simulink model "pmsm_FOC"  (R2018a)
settings: Solver=ode3  StartTime=0.0  StopTime=20  FixedStep=Ts  RelTol=1e-3  EnableMultiTasking=on
InitFcn:
  | % PMSM电机模型参数
  | P=8;
  | Ld=4.63e-4;
  | Lq=4.63e-4;
  | Flux_m=7.07e-3;
  | R=0.608;
  | J = 1.87e-3;
  | Beta=0;% 阻尼系数   (N s/m)
  | 
  | % 离散时间间隔
  | Ts = 1e-4;
  | 
  | % 观测器参数
  | w = 1000;
  | b = 500;
  | T = 0.01;
  | 
  | % TD微分跟踪器参数
  | tr=2000;
  | th = Ts*3;
  | 
  | % DOB转动惯量在线辨识参数
  | Jn = J
  | lamuda = 200
  | Te = 0.2
libraries: simulink x2, fuzblock x1
settings Model: Creator=www  LastModifiedBy=SPRain
settings SolverCC: AutoInsertRateTranBlk=on
settings DataIOCC: LimitDataPoints=on  SaveFormat=Array
settings OptimizationCC: ExpressionDepthLimit=2147483647  LifeSpan=inf
settings DebuggingCC: UnderspecifiedInitializationDetection=Classic  MergeDetectMultiDrivingBlocksExec=none  SolverPrmCheckMsg=warning  FcnCallInpInsideContextMsg=warning  StateNameClashWarn=warning  SFUnexpectedBacktrackingDiag=warning  SFNoUnconditionalDefaultTransitionDiag=warning  SFExecutionAtInitializationDiag=none
settings HardwareCC: ProdBitPerPointer=32  ProdBitPerSizeT=32  ProdBitPerPtrDiffT=32  ProdLargestAtomicFloat=None  ProdIntDivRoundTo=Undefined  ProdEndianess=Unspecified  ProdWordSize=32  ProdHWDeviceType=32-bit Generic
settings ModelReferenceCC: PropagateSignalLabelsOutOfModel=off
settings CodeAppCC: StateflowObjectComments=on
settings GRTTargetCC: TargetLangStandard=C89/C90 (ANSI)  GeneratePreprocessorConditionals=Disable all  CombineOutputUpdateFcns=off  GRTInterface=on
settings ConfigComp: CovMetricSettings=dw  CovHtmlReporting=on  CovSaveCumulativeToWorkspaceVar=on  CovSaveSingleToWorkspaceVar=on  CovExternalEMLEnable=off  CovSFcnEnable=off

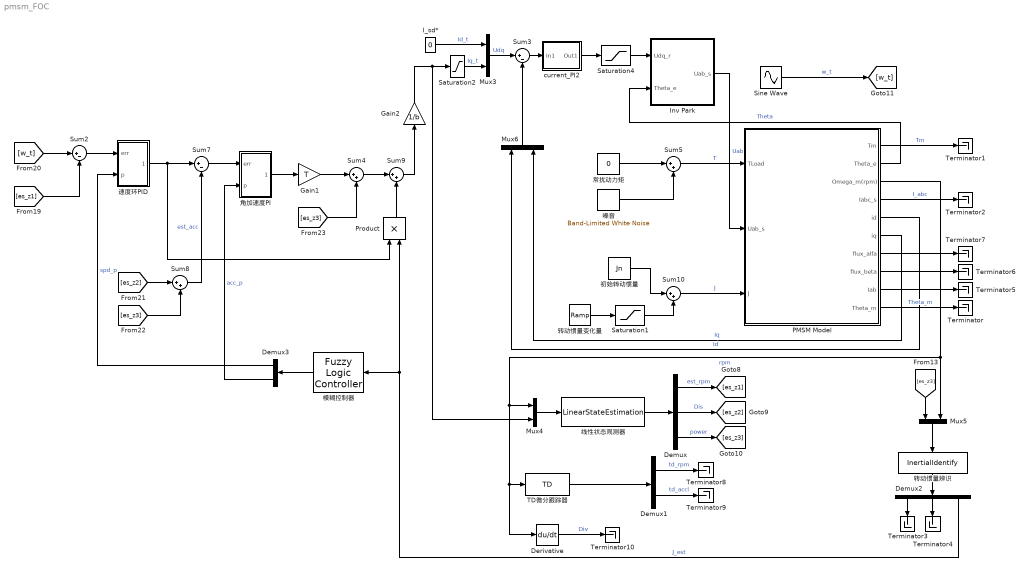
== system pmsm_FOC ==
  Demux : Demux  Outputs=3
  Demux1 : Demux  Outputs=2
  Demux2 : Demux  Outputs=3
  Demux3 : Demux  Outputs=2
  Derivative : Derivative
  Gain1 : Gain  Gain=T
  Gain2 : Gain  Gain=1/b
  I_sd* : Constant  Value=0
  Inv Park : Subsystem
  Mux{3..6} (4 alike) : Mux  Inputs=2
  PMSM Model : Subsystem
  Product : Product
  Saturation1 : Saturate  UpperLimit=0.02  LowerLimit=0
  Saturation2 : Saturate  UpperLimit=100  LowerLimit=-100
  Saturation4 : Saturate  UpperLimit=100  LowerLimit=-100
  Sine Wave : Sin  Amplitude=50  Frequency=5*pi  SampleTime=0
  Sum10 : Sum  Inputs=|++  SaturateOnIntegerOverflow=on  InputSameDT=on  OutDataTypeStr=Inherit: Same as first input
  Sum2 : Sum  Inputs=|+-
  Sum3 : Sum  Inputs=|+-
  Sum4 : Sum  Inputs=|++
  Sum5 : Sum  Inputs=|++  SaturateOnIntegerOverflow=on  InputSameDT=on  OutDataTypeStr=Inherit: Same as first input
  Sum7 : Sum  Inputs=|+-
  Sum8 : Sum  Inputs=|++  SaturateOnIntegerOverflow=on  InputSameDT=on  OutDataTypeStr=Inherit: Same as first input
  Sum9 : Sum  Inputs=|++
  TD微分跟踪器 : S-Function  FunctionName=TD  Parameters=tr,th,Ts  SFunctionDeploymentMode=off  EnableBusSupport=off
  Terminator{,1..10} (11 alike) : Terminator
  current_PI2 : Subsystem
  初始转动惯量 : Constant  Value=Jn
  噪音 : simulink/Sources/Band-Limited White Noise  Cov=[0.00001]  Ts=0.1  seed=[23341]
  常扰动力矩 : Constant  Value=0
  模糊控制器 : fuzblock/Fuzzy Logic  Controller  FIS='J_Fuzzy.fis'  OutputSampleNumber=101  DataType=double  FuzzifiedInputs=off  RuleFiringStrengths=off  RuleOutputs=off  AggregatedOutputs=off  SimulateUsing=Interpreted execution  OutOfRangeInputValueMessage=warning  NoRuleFiredMessage=warning  EmptyOutputFuzzySetMessage=warning
  线性状态观测器 : S-Function  FunctionName=LinearStateEstimation  Parameters=w,b,Ts,T  SFunctionDeploymentMode=off  EnableBusSupport=off
  角加速度PI : Subsystem
  转动惯量变化量 : simulink/Sources/Ramp  slope=0.002  start=5  InitialOutput=0
  转动惯量辨识 : S-Function  FunctionName=InertialIdentify  Parameters=lamuda,Ts,Te,Jn  SFunctionDeploymentMode=off  EnableBusSupport=off
  速度环PID : Subsystem
  wires:
  Saturation4/1 -> Inv Park/1(Udq_r)
  Inv Park/1(Uab_s) -> PMSM Model/2(Uab_s)  "Uab"
  I_sd*/1 -> Mux3/1  "Id_t"
  Mux3/1 -> Sum3/1  "Udq"
  Sum3/1 -> current_PI2/1(In1)
  current_PI2/1(Out1) -> Saturation4/1
  Mux6/1 -> Sum3/2
  PMSM Model/5(id) -> Mux6/1  "Id"
  PMSM Model/6(iq) -> Mux6/2  "Iq"
  PMSM Model/2(Theta_e) -> Inv Park/2(Theta_e)  "Theta"
  PMSM Model/1(Tm) -> Terminator1/1  "Tm"
  PMSM Model/4(Iabc_s) -> Terminator2/1  "I_abc"
  线性状态观测器/1 -> Demux/1
  Mux4/1 -> 线性状态观测器/1
  Demux/1 -> [es_z1]  "est_rpm"
  Demux/2 -> [es_z2]  "Dis"
  Demux/3 -> [es_z3]  "power"
  [es_z3] -> Mux5/1
  PMSM Model/3(Omega_m(rpm)) -> Mux4/1, Derivative/1, TD微分跟踪器/1, Mux5/2  "rpm"
  Sum5/1 -> PMSM Model/1(TLoad)  "T"
  常扰动力矩/1 -> Sum5/1
  噪音/1 -> Sum5/2
  TD微分跟踪器/1 -> Demux1/1
  Demux1/1 -> Terminator8/1  "td_rpm"
  Demux1/2 -> Terminator9/1  "td_accl"
  Derivative/1 -> Terminator10/1  "Div"
  Saturation2/1 -> Mux3/2  "Iq_t"
  [w_t] -> Sum2/1
  [es_z1] -> Sum2/2
  Sum2/1 -> 速度环PID/1(err)
  速度环PID/1(Out) -> Sum7/1, Product/1
  [es_z3] -> Sum8/2
  [es_z2] -> Sum8/1
  Sum8/1 -> Sum7/2  "est_acc"
  Sum7/1 -> 角加速度PI/1(err)
  Gain1/1 -> Sum4/1
  [es_z3] -> Sum4/2
  Gain2/1 -> Mux4/2, Saturation2/1
  Mux5/1 -> 转动惯量辨识/1
  转动惯量辨识/1 -> Demux2/1
  Demux2/3 -> 模糊控制器/1, Product/2  "J_est"
  Sum10/1 -> PMSM Model/3(J)  "J"
  初始转动惯量/1 -> Sum10/1
  模糊控制器/1 -> Demux3/1
  Demux3/1 -> 速度环PID/2(p)  "spd_p"
  Demux3/2 -> 角加速度PI/2(p)  "acc_p"
  Sine Wave/1 -> [w_t]  "w_t"
  转动惯量变化量/1 -> Saturation1/1
  角加速度PI/1(Out) -> Gain1/1
  Product/1 -> Sum9/2
  Sum4/1 -> Sum9/1
  Sum9/1 -> Gain2/1
  Saturation1/1 -> Sum10/2
  PMSM Model/10(Theta_m) -> Terminator/1  "Theta_m"
  Demux2/2 -> Terminator4/1
  Demux2/1 -> Terminator3/1
  PMSM Model/7(flux_alfa) -> Terminator7/1
  PMSM Model/8(flux_beta) -> Terminator6/1
  PMSM Model/9(Iab) -> Terminator5/1

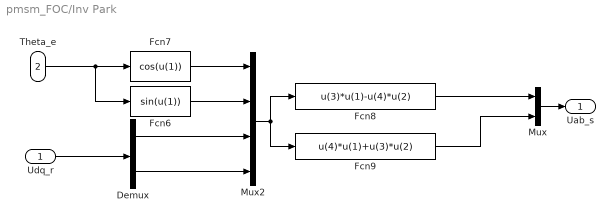
== system pmsm_FOC/Inv Park ==
  Udq_r : Inport
  Theta_e : Inport  Port=2
  Demux : Demux  Outputs=2
  Fcn6 : Fcn  Expr=sin(u(1))
  Fcn7 : Fcn  Expr=cos(u(1))
  Fcn8 : Fcn  Expr=u(3)*u(1)-u(4)*u(2)
  Fcn9 : Fcn  Expr=u(4)*u(1)+u(3)*u(2)
  Mux : Mux  Inputs=2
  Mux2 : Mux
  Uab_s : Outport
  wires:
  Theta_e/1 -> Fcn6/1, Fcn7/1
  Mux2/1 -> Fcn8/1, Fcn9/1
  Fcn6/1 -> Mux2/2
  Fcn7/1 -> Mux2/1
  Demux/1 -> Mux2/3
  Demux/2 -> Mux2/4
  Fcn9/1 -> Mux/2
  Fcn8/1 -> Mux/1
  Mux/1 -> Uab_s/1
  Udq_r/1 -> Demux/1

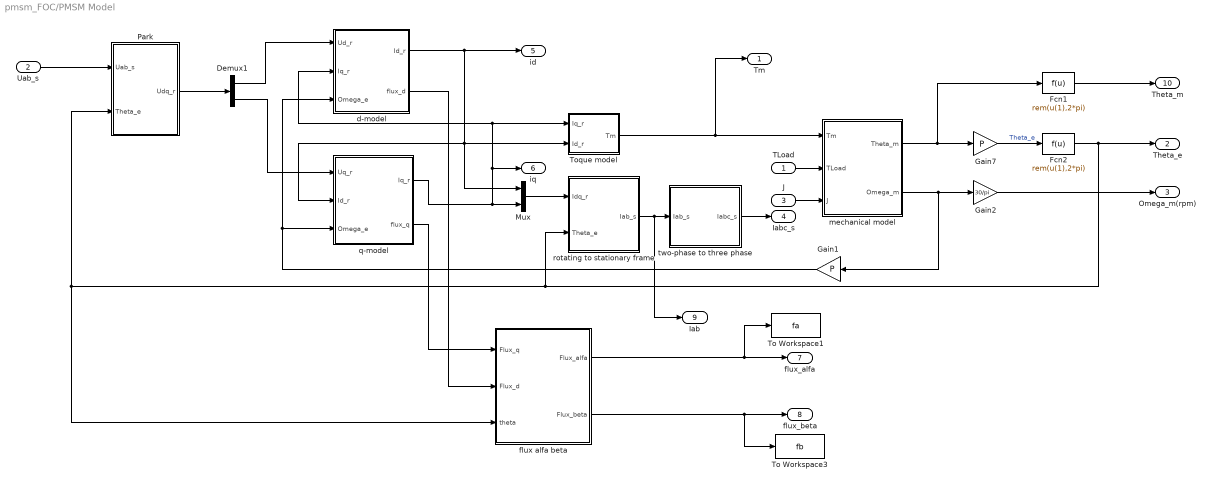
== system pmsm_FOC/PMSM Model ==
  TLoad : Inport
  Uab_s : Inport  Port=2
  J : Inport  Port=3
  Demux1 : Demux  Outputs=2
  Fcn1 : Fcn  Expr=rem(u(1),2*pi)
  Fcn2 : Fcn  Expr=rem(u(1),2*pi)
  Gain1 : Gain  Gain=P
  Gain2 : Gain  Gain=30/pi
  Gain7 : Gain  Gain=P
  Mux : Mux  Inputs=2
  Park : Subsystem
  To Workspace1 : ToWorkspace  VariableName=fa  SampleTime=-1
  To Workspace3 : ToWorkspace  VariableName=fb  SampleTime=-1
  Toque model : Subsystem
  d-model : Subsystem
  flux alfa beta : Subsystem
  mechanical model : Subsystem
  q-model : Subsystem
  rotating to stationary frame : Subsystem
  two-phase to three phase : Subsystem
  Tm : Outport
  Theta_e : Outport  Port=2
  Omega_m(rpm) : Outport  Port=3
  Iabc_s : Outport  Port=4
  id : Outport  Port=5
  iq : Outport  Port=6
  flux_alfa : Outport  Port=7
  flux_beta : Outport  Port=8
  Iab : Outport  Port=9
  Theta_m : Outport  Port=10
  wires:
  Gain7/1 -> Fcn2/1  "Theta_e"
  two-phase to three phase/1(Iabc_s) -> Iabc_s/1
  rotating to stationary frame/1(Iab_s) -> two-phase to three phase/1(Iab_s), Iab/1
  TLoad/1 -> mechanical model/2(TLoad)
  Toque model/1(Tm) -> Tm/1, mechanical model/1(Tm)
  mechanical model/1(Theta_m) -> Fcn1/1, Gain7/1
  mechanical model/2(Omega_m) -> Gain1/1, Gain2/1
  Mux/1 -> rotating to stationary frame/1(Idq_r)
  q-model/1(Iq_r) -> d-model/2(Iq_r), Toque model/1(Iq_r), iq/1, Mux/2
  d-model/1(Id_r) -> id/1, q-model/2(Id_r), Mux/1, Toque model/2(Id_r)
  Demux1/2 -> q-model/1(Uq_r)
  Demux1/1 -> d-model/1(Ud_r)
  Park/1(Udq_r) -> Demux1/1
  Gain1/1 -> q-model/3(Omega_e), d-model/3(Omega_e)
  Fcn2/1 -> Theta_e/1, rotating to stationary frame/2(Theta_e), flux alfa beta/3(theta), Park/2(Theta_e)
  d-model/2(flux_d) -> flux alfa beta/2(Flux_d)
  q-model/2(flux_q) -> flux alfa beta/1(Flux_q)
  flux alfa beta/1(Flux_alfa) -> flux_alfa/1, To Workspace1/1
  flux alfa beta/2(Flux_beta) -> flux_beta/1, To Workspace3/1
  Uab_s/1 -> Park/1(Uab_s)
  Gain2/1 -> Omega_m(rpm)/1
  J/1 -> mechanical model/3(J)
  Fcn1/1 -> Theta_m/1

== system pmsm_FOC/current_PI2 ==
  In1 : Inport
  Gain : Gain  Gain=1.3
  Gain1 : Gain  Gain=0.05
  Integrator : Integrator
  Sum1 : Sum  Inputs=|++
  Out1 : Outport
  wires:
  Gain/1 -> Integrator/1, Sum1/1
  Integrator/1 -> Gain1/1
  Gain1/1 -> Sum1/2
  In1/1 -> Gain/1
  Sum1/1 -> Out1/1

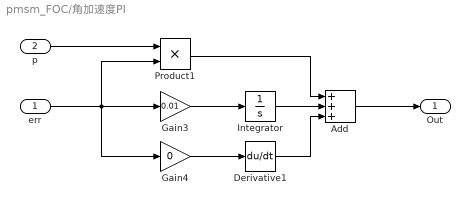
== system pmsm_FOC/角加速度PI ==
  err : Inport
  p : Inport  Port=2
  Add : Sum  Inputs=+++
  Derivative1 : Derivative
  Gain3 : Gain  Gain=0.01
  Gain4 : Gain  Gain=0
  Integrator : Integrator
  Product1 : Product
  Out : Outport
  wires:
  Add/1 -> Out/1
  err/1 -> Gain4/1, Product1/2, Gain3/1
  Derivative1/1 -> Add/3
  p/1 -> Product1/1
  Product1/1 -> Add/1
  Integrator/1 -> Add/2
  Gain3/1 -> Integrator/1
  Gain4/1 -> Derivative1/1

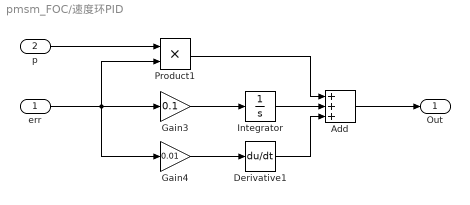
== system pmsm_FOC/速度环PID ==
  err : Inport
  p : Inport  Port=2
  Add : Sum  Inputs=+++
  Derivative1 : Derivative
  Gain3 : Gain  Gain=0.1
  Gain4 : Gain  Gain=0.01
  Integrator : Integrator
  Product1 : Product
  Out : Outport
  wires:
  Gain4/1 -> Derivative1/1
  Gain3/1 -> Integrator/1
  Integrator/1 -> Add/2
  Product1/1 -> Add/1
  p/1 -> Product1/1
  Derivative1/1 -> Add/3
  err/1 -> Gain3/1, Product1/2, Gain4/1
  Add/1 -> Out/1

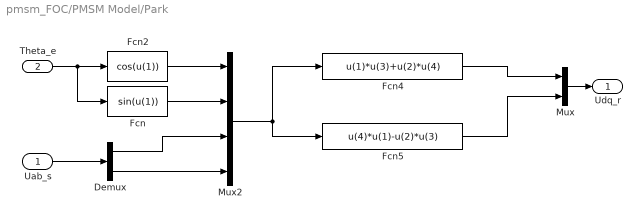
== system pmsm_FOC/PMSM Model/Park ==
  Uab_s : Inport
  Theta_e : Inport  Port=2
  Demux : Demux  Outputs=2
  Fcn : Fcn  Expr=sin(u(1))
  Fcn2 : Fcn  Expr=cos(u(1))
  Fcn4 : Fcn  Expr=u(1)*u(3)+u(2)*u(4)
  Fcn5 : Fcn  Expr=u(4)*u(1)-u(2)*u(3)
  Mux : Mux  Inputs=2
  Mux2 : Mux
  Udq_r : Outport
  wires:
  Uab_s/1 -> Demux/1
  Mux/1 -> Udq_r/1
  Theta_e/1 -> Fcn/1, Fcn2/1
  Fcn5/1 -> Mux/2
  Fcn4/1 -> Mux/1
  Mux2/1 -> Fcn5/1, Fcn4/1
  Demux/2 -> Mux2/4
  Demux/1 -> Mux2/3
  Fcn/1 -> Mux2/2
  Fcn2/1 -> Mux2/1

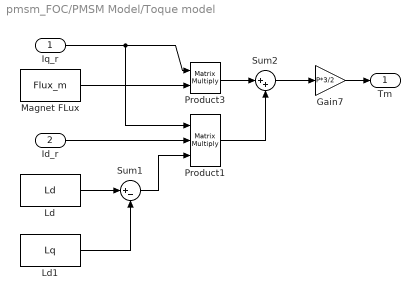
== system pmsm_FOC/PMSM Model/Toque model ==
  Iq_r : Inport
  Id_r : Inport  Port=2
  Gain7 : Gain  Gain=P*3/2
  Ld : Constant  Value=Ld
  Ld1 : Constant  Value=Lq
  Magnet FLux : Constant  Value=Flux_m
  Product1 : Product  Inputs=3  Multiplication=Matrix(*)  RndMeth=Zero
  Product3 : Product  Multiplication=Matrix(*)  RndMeth=Zero
  Sum1 : Sum  Inputs=|+-
  Sum2 : Sum  Inputs=|++
  Tm : Outport
  wires:
  Product1/1 -> Sum2/2
  Sum1/1 -> Product1/3
  Id_r/1 -> Product1/2
  Ld1/1 -> Sum1/2
  Ld/1 -> Sum1/1
  Sum2/1 -> Gain7/1
  Product3/1 -> Sum2/1
  Magnet FLux/1 -> Product3/2
  Gain7/1 -> Tm/1
  Iq_r/1 -> Product1/1, Product3/1

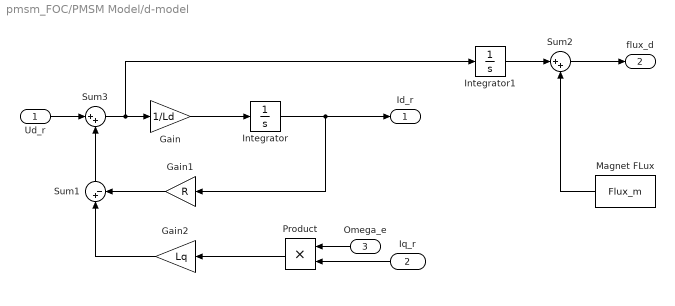
== system pmsm_FOC/PMSM Model/d-model ==
  Ud_r : Inport
  Iq_r : Inport  Port=2
  Omega_e : Inport  Port=3
  Gain : Gain  Gain=1/Ld
  Gain1 : Gain  Gain=R
  Gain2 : Gain  Gain=Lq
  Integrator : Integrator
  Integrator1 : Integrator
  Magnet FLux : Constant  Value=Flux_m
  Product : Product  RndMeth=Zero
  Sum1 : Sum  Inputs=|+-
  Sum2 : Sum  Inputs=|++
  Sum3 : Sum  Inputs=|++
  Id_r : Outport
  flux_d : Outport  Port=2
  wires:
  Ud_r/1 -> Sum3/1
  Iq_r/1 -> Product/2
  Omega_e/1 -> Product/1
  Product/1 -> Gain2/1
  Gain2/1 -> Sum1/1
  Sum1/1 -> Sum3/2
  Gain1/1 -> Sum1/2
  Integrator/1 -> Id_r/1, Gain1/1
  Gain/1 -> Integrator/1
  Sum3/1 -> Gain/1, Integrator1/1
  Integrator1/1 -> Sum2/1
  Magnet FLux/1 -> Sum2/2
  Sum2/1 -> flux_d/1

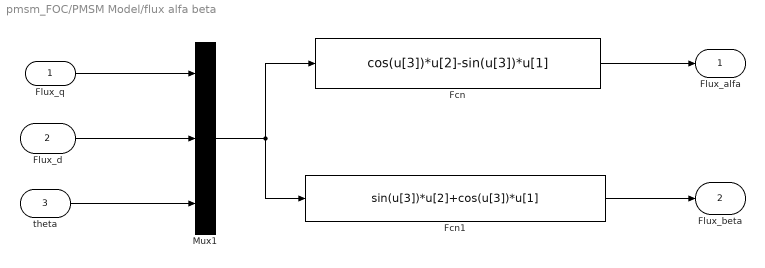
== system pmsm_FOC/PMSM Model/flux alfa beta ==
  Flux_q : Inport
  Flux_d : Inport  Port=2
  theta : Inport  Port=3
  Fcn : Fcn  Expr=cos(u[3])*u[2]-sin(u[3])*u[1]
  Fcn1 : Fcn  Expr=sin(u[3])*u[2]+cos(u[3])*u[1]
  Mux1 : Mux  Inputs=3
  Flux_alfa : Outport
  Flux_beta : Outport  Port=2
  wires:
  Mux1/1 -> Fcn/1, Fcn1/1
  Flux_q/1 -> Mux1/1
  Fcn/1 -> Flux_alfa/1
  Flux_d/1 -> Mux1/2
  Fcn1/1 -> Flux_beta/1
  theta/1 -> Mux1/3

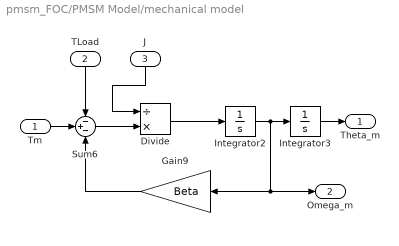
== system pmsm_FOC/PMSM Model/mechanical model ==
  Tm : Inport
  TLoad : Inport  Port=2
  J : Inport  Port=3
  Divide : Product  Inputs=/*
  Gain9 : Gain  Gain=Beta
  Integrator2 : Integrator
  Integrator3 : Integrator
  Sum6 : Sum  Inputs=-+-
  Theta_m : Outport
  Omega_m : Outport  Port=2
  wires:
  TLoad/1 -> Sum6/1
  Gain9/1 -> Sum6/3
  Tm/1 -> Sum6/2
  Integrator3/1 -> Theta_m/1
  Integrator2/1 -> Omega_m/1, Gain9/1, Integrator3/1
  Divide/1 -> Integrator2/1
  Sum6/1 -> Divide/2
  J/1 -> Divide/1

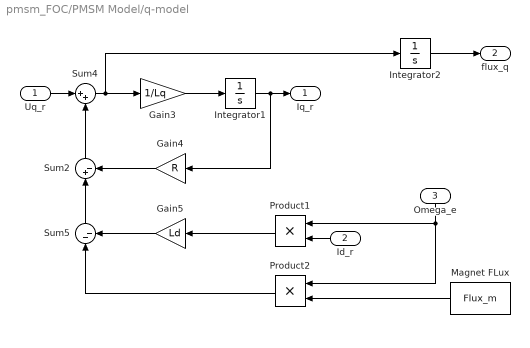
== system pmsm_FOC/PMSM Model/q-model ==
  Uq_r : Inport
  Id_r : Inport  Port=2
  Omega_e : Inport  Port=3
  Gain3 : Gain  Gain=1/Lq
  Gain4 : Gain  Gain=R
  Gain5 : Gain  Gain=Ld
  Integrator1 : Integrator
  Integrator2 : Integrator
  Magnet FLux : Constant  Value=Flux_m
  Product1 : Product  RndMeth=Zero
  Product2 : Product  RndMeth=Zero
  Sum2 : Sum  Inputs=|+-
  Sum4 : Sum  Inputs=|++
  Sum5 : Sum  Inputs=|--
  Iq_r : Outport
  flux_q : Outport  Port=2
  wires:
  Id_r/1 -> Product1/2
  Omega_e/1 -> Product2/1, Product1/1
  Magnet FLux/1 -> Product2/2
  Product2/1 -> Sum5/1
  Product1/1 -> Gain5/1
  Sum5/1 -> Sum2/1
  Gain5/1 -> Sum5/2
  Gain4/1 -> Sum2/2
  Integrator1/1 -> Iq_r/1, Gain4/1
  Gain3/1 -> Integrator1/1
  Sum4/1 -> Gain3/1, Integrator2/1
  Uq_r/1 -> Sum4/1
  Sum2/1 -> Sum4/2
  Integrator2/1 -> flux_q/1

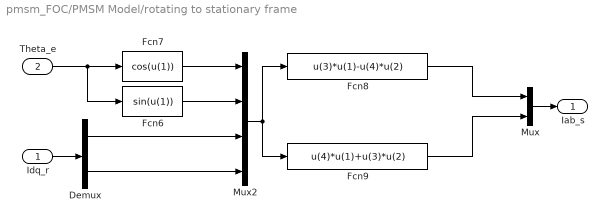
== system pmsm_FOC/PMSM Model/rotating to stationary frame ==
  Idq_r : Inport
  Theta_e : Inport  Port=2
  Demux : Demux  Outputs=2
  Fcn6 : Fcn  Expr=sin(u(1))
  Fcn7 : Fcn  Expr=cos(u(1))
  Fcn8 : Fcn  Expr=u(3)*u(1)-u(4)*u(2)
  Fcn9 : Fcn  Expr=u(4)*u(1)+u(3)*u(2)
  Mux : Mux  Inputs=2
  Mux2 : Mux
  Iab_s : Outport
  wires:
  Idq_r/1 -> Demux/1
  Mux/1 -> Iab_s/1
  Fcn8/1 -> Mux/1
  Fcn9/1 -> Mux/2
  Demux/2 -> Mux2/4
  Demux/1 -> Mux2/3
  Fcn7/1 -> Mux2/1
  Fcn6/1 -> Mux2/2
  Mux2/1 -> Fcn9/1, Fcn8/1
  Theta_e/1 -> Fcn7/1, Fcn6/1

== system pmsm_FOC/PMSM Model/two-phase to three phase ==
  Iab_s : Inport
  Fcn10 : Fcn  Expr=u(1)
  Fcn11 : Fcn  Expr=-0.5*u(1)+sqrt(3)/2*u(2)
  Fcn12 : Fcn  Expr=-0.5*u(1)-sqrt(3)/2*u(2)
  Mux2 : Mux  Inputs=3
  Iabc_s : Outport
  wires:
  Mux2/1 -> Iabc_s/1
  Fcn12/1 -> Mux2/3
  Fcn10/1 -> Mux2/1
  Fcn11/1 -> Mux2/2
  Iab_s/1 -> Fcn10/1, Fcn11/1, Fcn12/1
